simulink model "Quadraturmodulator"  (Simulink 8.5)
settings: Solver=FixedStepDiscrete  StartTime=0  StopTime=inf  RelTol=1e-3
undefined symbols (not defined in the file): fs
libraries: dspsrcs4 x4, dspmlti4 x2, simulink x1
settings Model: Creator=schwall  LastModifiedBy=wunsch  CovSFcnEnable=off
settings DataIOCC: LimitDataPoints=off  SaveOutput=off  SignalLogging=off  SaveTime=off
settings DebuggingCC: SolverPrmCheckMsg=warning  FcnCallInpInsideContextMsg=UseLocalSettings

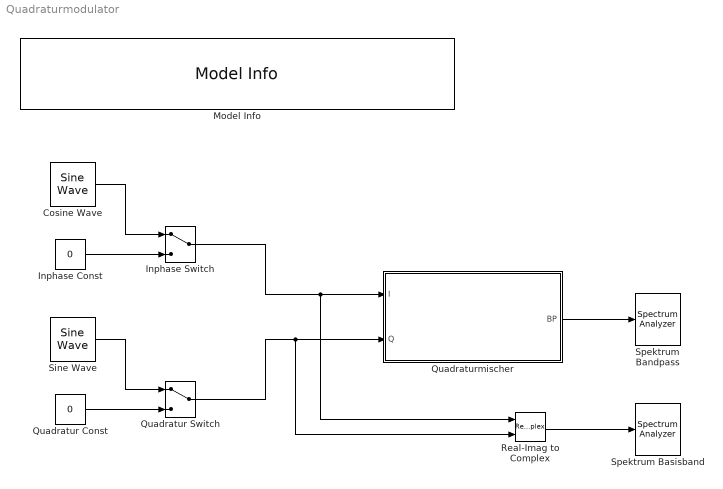
== system Quadraturmodulator ==
  Cosine Wave : dspsrcs4/Sine Wave  Amplitude=1  Frequency=20000  Phase=pi/2  SampleMode=Discrete  OutComplex=Real  CompMethod=Trigonometric fcn  TableSize=Speed  SampleTime=1/fs*10  SamplesPerFrame=1  ResetState=Restart at time zero  dataType=double  wordLen=16  udDataType=sfix(16)  fracBitsMode=Best precision  numFracBits=15  OutDataTypeStr=double  LastOutDataTypeStr=double
  Inphase Const : Constant  Value=0
  Inphase Switch : ManualSwitch
  Model Info : simulink/Model-Wide Utilities/Model Info  BlockCM=None  Frame=on  DisplayStringWithTags=|  HorizontalTextAlignment=Left  LeftAlignmentValue=0.02  SourceBlockDiagram=Quadraturmodulator  TagMaxNumber=20
      | Demo Quadraturmodulator
      | Vorlesung Nachrichtentechnik II
      | Institut fuer Nachrichtentechnik (CEL)
  Quadratur Const : Constant  Value=0
  Quadratur Switch : ManualSwitch
  Quadraturmischer : Subsystem  mask(Quadraturmischer-Modell){fs=1e6, fc=200e3, Ai=1, fi=0, phii=0, Aq=1, fq=0, phiq=0}
      mask prompts: fs "Abtastfrequenz [Hz]"; fc "Traegerfrequenz [Hz]"; Ai "Amplitude Inphase (Ai)"; fi "Frequenz-Offset Inphase (fi) [Hz]"; phii "Phasenverschiebung Inphase (phii) [rad]"; Aq "Amplitude Quadratur (Aq)"; fq "Frequenz-Offset Quadratur (fq) [Hz]"; phiq "Phasenverschiebung Quadratur (phiq) [rad]"
      mask help:
      | s(t) = I(t) Ai cos(2pi(fc+fi)t+phii) - Q(t) Aq sin(2pi(fc+fq)t+phiq)
      | (ggf. Neustart nach Parameteraenderung noetig)
      mask init:
      | assignin('base','fs',fs)
      mask Display:
      | port_label('output', 1, 'BP')
      | port_label('input', 1, 'I')
      | port_label('input', 2, 'Q')
      | disp('Quadraturmodulator')
  Real-Imag to Complex : RealImagToComplex
  Sine Wave : dspsrcs4/Sine Wave  Amplitude=1  Frequency=20000  Phase=0  SampleMode=Discrete  OutComplex=Real  CompMethod=Trigonometric fcn  TableSize=Speed  SampleTime=1/fs*10  SamplesPerFrame=1  ResetState=Restart at time zero  dataType=double  wordLen=16  udDataType=sfix(16)  fracBitsMode=Best precision  numFracBits=15  OutDataTypeStr=double  LastOutDataTypeStr=double
  Spektrum Bandpass : SpectrumAnalyzer
  Spektrum Basisband : SpectrumAnalyzer
  wires:
  Quadraturmischer/1(BP) -> Spektrum Bandpass/1
  Real-Imag to Complex/1 -> Spektrum Basisband/1
  Inphase Const/1 -> Inphase Switch/2
  Quadratur Const/1 -> Quadratur Switch/2
  Quadratur Switch/1 -> Quadraturmischer/2(Q), Real-Imag to Complex/2
  Inphase Switch/1 -> Quadraturmischer/1(I), Real-Imag to Complex/1
  Sine Wave/1 -> Quadratur Switch/1
  Cosine Wave/1 -> Inphase Switch/1

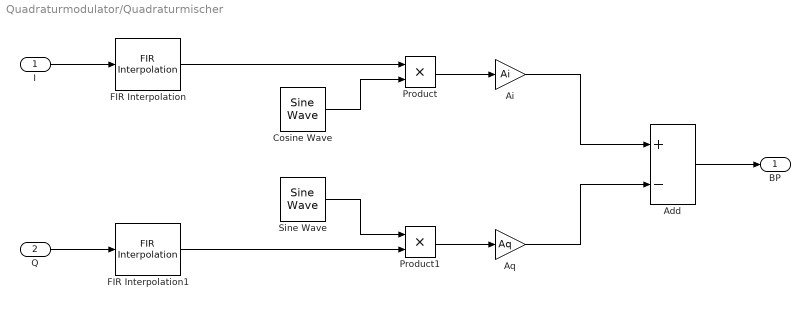
== system Quadraturmodulator/Quadraturmischer ==
  I : Inport
  Q : Inport  Port=2
  Add : Sum  Inputs=+-
  Ai : Gain  Gain=Ai
  Aq : Gain  Gain=Aq
  Cosine Wave : dspsrcs4/Sine Wave  Amplitude=1  Frequency=fc  Phase=phii  SampleMode=Discrete  OutComplex=Real  CompMethod=Trigonometric fcn  TableSize=Speed  SampleTime=1/fs  SamplesPerFrame=1  ResetState=Restart at time zero  dataType=double  wordLen=16  udDataType=sfix(16)  fracBitsMode=Best precision  numFracBits=15  OutDataTypeStr=double  LastOutDataTypeStr=double
  FIR Interpolation : dspmlti4/FIR Interpolation  h=fir1(40,1/20)  L=10  framing=Allow multirate processing  outputBufInitCond=0  firstCoeffDataTypeStr=Inherit: Same word length as input  firstCoeffLastDataTypeStr=Inherit: Same word length as input  firstCoeffMin=[]  firstCoeffMax=[]  outputDataTypeStr=Inherit: Same as accumulator  outputLastDataTypeStr=Inherit: Same as accumulator  outputMin=[]  outputMax=[]  roundingMode=Floor  overflowMode=off  FilterSource=Specify via dialog  FilterObject=Hm_firinterp
  FIR Interpolation1 : dspmlti4/FIR Interpolation  h=fir1(40,1/20)  L=10  framing=Allow multirate processing  outputBufInitCond=0  firstCoeffDataTypeStr=Inherit: Same word length as input  firstCoeffLastDataTypeStr=Inherit: Same word length as input  firstCoeffMin=[]  firstCoeffMax=[]  outputDataTypeStr=Inherit: Same as accumulator  outputLastDataTypeStr=Inherit: Same as accumulator  outputMin=[]  outputMax=[]  roundingMode=Floor  overflowMode=off  FilterSource=Specify via dialog  FilterObject=Hm_firinterp
  Product : Product  RndMeth=Zero
  Product1 : Product  RndMeth=Zero
  Sine Wave : dspsrcs4/Sine Wave  Amplitude=1  Frequency=fc  Phase=pi/2+phiq+pi  SampleMode=Discrete  OutComplex=Real  CompMethod=Trigonometric fcn  TableSize=Speed  SampleTime=1/fs  SamplesPerFrame=1  ResetState=Restart at time zero  dataType=double  wordLen=16  udDataType=sfix(16)  fracBitsMode=Best precision  numFracBits=15  OutDataTypeStr=double  LastOutDataTypeStr=double
  BP : Outport
  wires:
  Product/1 -> Ai/1
  Product1/1 -> Aq/1
  I/1 -> FIR Interpolation/1
  Add/1 -> BP/1
  Q/1 -> FIR Interpolation1/1
  Ai/1 -> Add/1
  Aq/1 -> Add/2
  FIR Interpolation/1 -> Product/1
  FIR Interpolation1/1 -> Product1/2
  Cosine Wave/1 -> Product/2
  Sine Wave/1 -> Product1/1
